simulink model "TestDebitMoteurNew"  (Simulink 6.5)
settings: Solver=FixedStepDiscrete  StartTime=0.0  StopTime=SimuPumpStop  FixedStep=0.1  RelTol=1e-6
undefined symbols (not defined in the file): PcolTest, PumpedTest, RegimeTest, TempsTest, TimePumpedTest, x
settings Model: Creator=a030141  LastModifiedBy=Zeus
settings DataIOCC: SignalLoggingName=sigsOut
settings DebuggingCC: SolverPrmCheckMsg=none  MultiTaskDSMMsg=warning  MultiTaskCondExecSysMsg=none  StrictBusMsg=None
settings HardwareCC: TargetUnknown=on
settings RTWCC: IncludeERTFirstTime=on

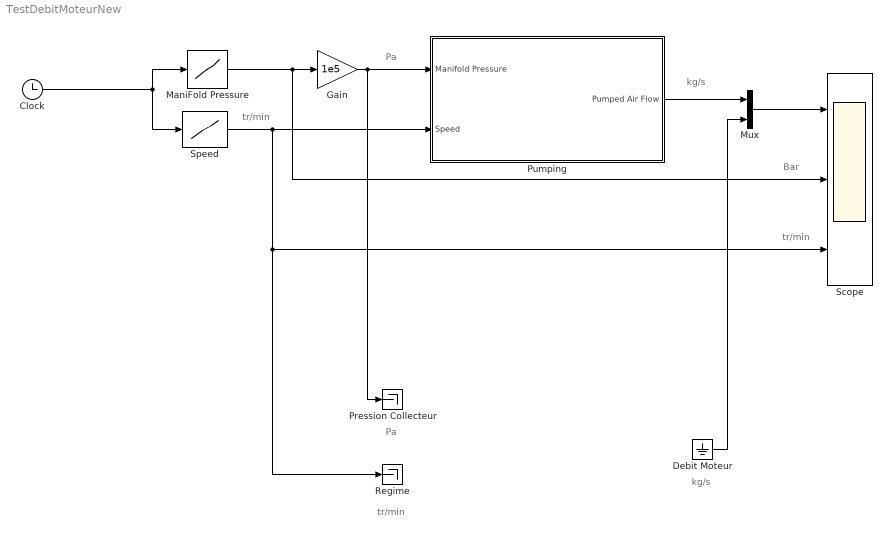
== system TestDebitMoteurNew ==
  note: kg/s
  note: Pa
  note: Bar
  note: tr/min
  note: tr/min
  note: Pa
  note: tr/min
  note: kg/s
  Clock : Clock
      settings: Decimation=10
  Debit Moteur : Ground
  Gain : Gain  Gain=1e5  SaturateOnIntegerOverflow=on
  ManiFold Pressure : Lookup  InputValues=TempsTest  OutputValues=PcolTest  LookUpMeth=Interpolation-Extrapolation  OutDataType=sfix(16)  OutScaling=2^0  SaturateOnIntegerOverflow=on  SampleTime=-1  LUTDesignTableMode=Redesign Table  LUTDesignDataSource=Block Dialog  LUTDesignFunctionName=sqrt(x)  LUTDesignUseExistingBP=on  LUTDesignRelError=0.01  LUTDesignAbsError=1e-6  RndMeth=Floor
      settings: LockScale=off
  Mux : Mux  Inputs=2
  Pression Collecteur : Terminator
  Pumping : Subsystem
  Regime : Terminator
  Scope : Scope  NumInputPorts=3
      settings: TimeRange=596.5  YMin=-5~-5~-5  YMax=5~5~5
  Speed : Lookup  InputValues=TempsTest  OutputValues=RegimeTest  LookUpMeth=Interpolation-Extrapolation  OutDataType=sfix(16)  OutScaling=2^0  SaturateOnIntegerOverflow=on  SampleTime=-1  LUTDesignTableMode=Redesign Table  LUTDesignDataSource=Block Dialog  LUTDesignFunctionName=sqrt(x)  LUTDesignUseExistingBP=on  LUTDesignRelError=0.01  LUTDesignAbsError=1e-6  RndMeth=Floor
      settings: LockScale=off
  wires:
  Speed/1 -> Scope/3, Regime/1, Pumping/2(Speed)
  Clock/1 -> ManiFold Pressure/1, Speed/1
  ManiFold Pressure/1 -> Gain/1, Scope/2
  Gain/1 -> Pression Collecteur/1, Pumping/1(Manifold Pressure)
  Mux/1 -> Scope/1
  Debit Moteur/1 -> Mux/2
  Pumping/1(Pumped Air Flow) -> Mux/1

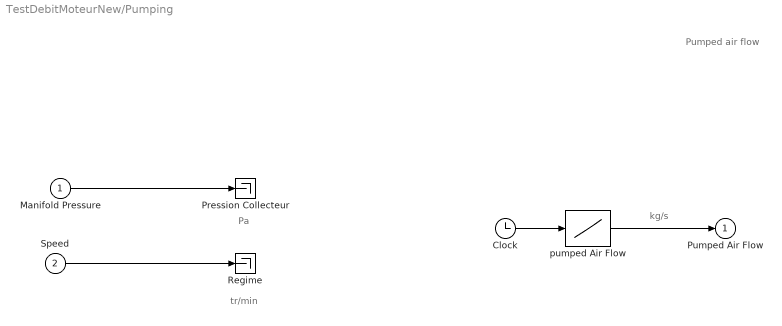
== system TestDebitMoteurNew/Pumping ==
  note: Pumped air flow
  note: kg/s
  note: Pa
  note: tr/min
  Manifold Pressure : Inport
  Speed : Inport  Port=2
  Clock : Clock
      settings: Decimation=10
  Pression Collecteur : Terminator
  Regime : Terminator
  pumped Air Flow : Lookup  InputValues=TimePumpedTest  OutputValues=PumpedTest  LookUpMeth=Interpolation-Extrapolation  OutDataType=sfix(16)  OutScaling=2^0  SaturateOnIntegerOverflow=on  SampleTime=-1  LUTDesignTableMode=Redesign Table  LUTDesignDataSource=Block Dialog  LUTDesignFunctionName=sqrt(x)  LUTDesignUseExistingBP=on  LUTDesignRelError=0.01  LUTDesignAbsError=1e-6  RndMeth=Floor
      settings: LockScale=off
  Pumped Air Flow : Outport
  wires:
  Manifold Pressure/1 -> Pression Collecteur/1
  Speed/1 -> Regime/1
  pumped Air Flow/1 -> Pumped Air Flow/1
  Clock/1 -> pumped Air Flow/1
